simulink model "DC_Drive"  (R2021a)
settings: Solver=VariableStepAuto  StartTime=0.0  StopTime=13  MaxStep=1e-5  RelTol=1e-3
undefined symbols (not defined in the file): sigbuilder_block
libraries: spsMeanLib x6, simulink_extras x5, spsSawtoothGeneratorLib x4, spsTriangleGeneratorLib x2
settings Model: SimulationMode=accelerator  Creator=AHMED  LastModifiedBy=AHMED

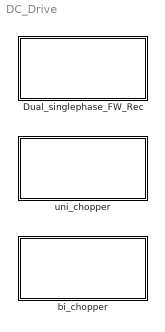
== system DC_Drive ==
  Dual_singlephase_FW_Rec : Subsystem
  bi_chopper : Subsystem
  uni_chopper : Subsystem

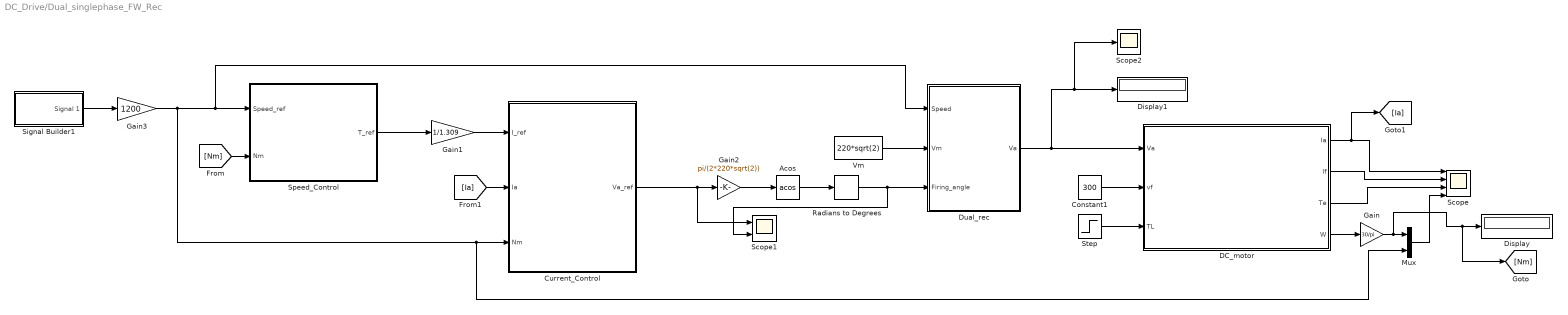
== system DC_Drive/Dual_singlephase_FW_Rec ==
  Acos : Trigonometry  Operator=acos
  Constant1 : Constant  Value=300
  Current_Control : Subsystem
  DC_motor : Subsystem  mask{Ra=0.6, La=12e-3, Rf=240, Lf=120, J=0.05, K=1.309}
  Display : Display
  Display1 : Display
  Dual_rec : Subsystem
  Gain : Gain  Gain=30/pi
  Gain1 : Gain  Gain=1/1.309
  Gain2 : Gain  Gain=pi/(2*220*sqrt(2))
  Gain3 : Gain  Gain=1200
  Mux : Mux  Inputs=2
  Radians to Degrees : simulink_extras/Transformations/Radians to Degrees
  Scope : Scope  NumInputPorts=4
  Scope1 : Scope  NumInputPorts=2
  Scope2 : Scope
  Signal Builder1 : Subsystem  Tag=STV Subsys  LoadFcn=sigbuilder_block('load');  StartFcn=sigbuilder_block('start');  StopFcn=sigbuilder_block('stop');  ClipboardFcn=sigbuilder_block('clipboard');  mask(Sigbuilder block){tuvar=[0:10]}
      mask help: Simulink:masks:SigbuilderBlock_MD
      mask init:
      | if ~strcmp(get_param(bdroot(gcbh),'SimulationStatus'),'stopped') tuvar = sigbuilder_block('maskInit'); end
      settings: CopyFcn=sigbuilder_block('copy');  DeleteFcn=sigbuilder_block('delete');  ModelCloseFcn=sigbuilder_block('modelClose');  PreSaveFcn=sigbuilder_block('preSave');  PauseFcn=sigbuilder_block('pause');  ContinueFcn=sigbuilder_block('continue');  NameChangeFcn=sigbuilder_block('namechange');  OpenFcn=sigbuilder_block('open',[5.4 30 1141.2 522.6 ]);  CloseFcn=sigbuilder_block('close');
      mask Display: plot(0, 0, 100, 100,[2, 2, 32, 32, 2], [68, 8, 8, 68, 68],[32, 2], [38, 38], [32, 19, 2],[53, 60, 44], [32, 17, 17, 2],[16, 16, 31, 31]);txt = getActiveGroup(gcbh);text(2, 100, txt,'verticalAlignment', 'top');
  Speed_Control : Subsystem
  Step : Step  Time=2.25  After=5  SampleTime=0
  Vm : Constant  Value=220*sqrt(2)
  wires:
  Mux/1 -> Scope/4
  Dual_rec/1(Va) -> Scope2/1, Display1/1, DC_motor/1(Va)
  Gain3/1 -> Mux/2, Current_Control/3(Nm), Dual_rec/1(Speed), Speed_Control/1(Speed_ref)
  Current_Control/1(Va_ref) -> Scope1/1, Gain2/1
  Constant1/1 -> DC_motor/2(vf)
  Vm/1 -> Dual_rec/2(Vm)
  DC_motor/2(If) -> Scope/2
  DC_motor/3(Te) -> Scope/3
  Radians to Degrees/1 -> Scope1/2, Dual_rec/3(Firing_angle)
  DC_motor/4(W) -> Gain/1
  Signal Builder1/1(Signal 1) -> Gain3/1
  Gain/1 -> [Nm], Display/1, Mux/1
  DC_motor/1(Ia) -> [Ia], Scope/1
  Acos/1 -> Radians to Degrees/1
  [Nm] -> Speed_Control/2(Nm)
  Speed_Control/1(T_ref) -> Gain1/1
  Gain1/1 -> Current_Control/1(I_ref)
  [Ia] -> Current_Control/2(Ia)
  Step/1 -> DC_motor/3(TL)
  Gain2/1 -> Acos/1

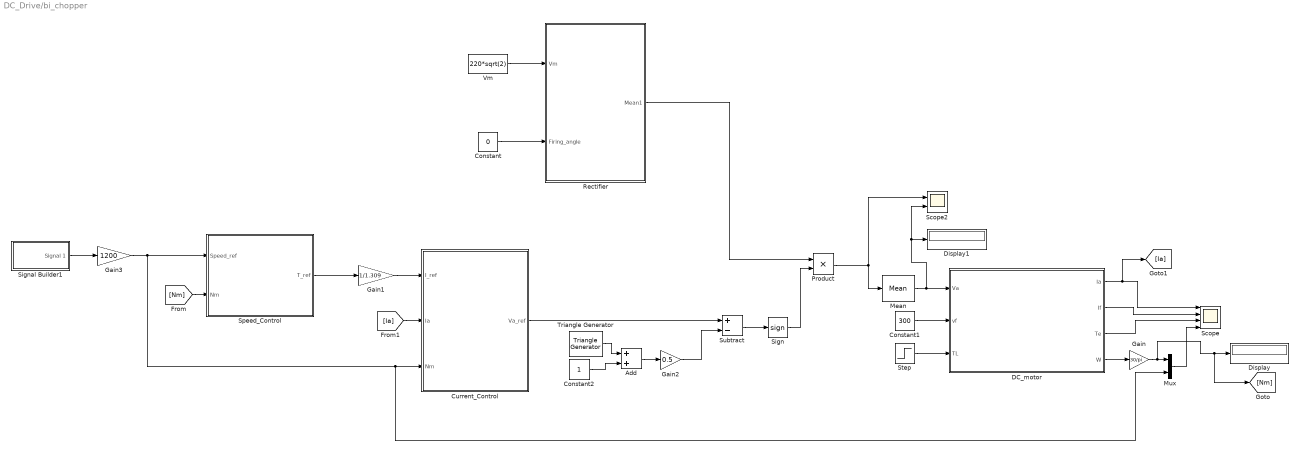
== system DC_Drive/bi_chopper ==
  Add : Sum
  Constant : Constant  Value=0
  Constant1 : Constant  Value=300
  Constant2 : Constant
  Current_Control : Subsystem
  DC_motor : Subsystem  mask{Ra=0.6, La=12e-3, Rf=240, Lf=120, J=0.05, K=1.309}
  Display : Display
  Display1 : Display
  Gain : Gain  Gain=30/pi
  Gain1 : Gain  Gain=1/1.309
  Gain2 : Gain  Gain=0.5
  Gain3 : Gain  Gain=1200
  Mean : spsMeanLib/Mean  Freq=50  Vinit=0  Ts=0
  Mux : Mux  Inputs=2
  Product : Product
  Rectifier : Subsystem
  Scope : Scope  NumInputPorts=4
  Scope2 : Scope  NumInputPorts=2
  Sign : Signum
  Signal Builder1 : Subsystem  Tag=STV Subsys  LoadFcn=sigbuilder_block('load');  StartFcn=sigbuilder_block('start');  StopFcn=sigbuilder_block('stop');  ClipboardFcn=sigbuilder_block('clipboard');  mask(Sigbuilder block){tuvar=[0:10]}
      mask help: Simulink:masks:SigbuilderBlock_MD
      mask init:
      | if ~strcmp(get_param(bdroot(gcbh),'SimulationStatus'),'stopped') tuvar = sigbuilder_block('maskInit'); end
      settings: CopyFcn=sigbuilder_block('copy');  DeleteFcn=sigbuilder_block('delete');  ModelCloseFcn=sigbuilder_block('modelClose');  PreSaveFcn=sigbuilder_block('preSave');  PauseFcn=sigbuilder_block('pause');  ContinueFcn=sigbuilder_block('continue');  NameChangeFcn=sigbuilder_block('namechange');  OpenFcn=sigbuilder_block('open',[5.4 30 1141.2 522.6 ]);  CloseFcn=sigbuilder_block('close');
      mask Display: plot(0, 0, 100, 100,[2, 2, 32, 32, 2], [68, 8, 8, 68, 68],[32, 2], [38, 38], [32, 19, 2],[53, 60, 44], [32, 17, 17, 2],[16, 16, 31, 31]);txt = getActiveGroup(gcbh);text(2, 100, txt,'verticalAlignment', 'top');
  Speed_Control : Subsystem
  Step : Step  Time=2.25  After=5  SampleTime=0
  Subtract : Sum  Inputs=+-
  Triangle Generator : spsTriangleGeneratorLib/Triangle Generator  Freq=1e3  Phase=90  Ts=0
  Vm : Constant  Value=220*sqrt(2)
  wires:
  Mean/1 -> DC_motor/1(Va), Scope2/2, Display1/1
  Add/1 -> Gain2/1
  Constant2/1 -> Add/2
  Triangle Generator/1 -> Add/1
  Constant/1 -> Rectifier/2(Firing_angle)
  Mux/1 -> Scope/4
  Product/1 -> Mean/1, Scope2/1
  Gain3/1 -> Mux/2, Current_Control/3(Nm), Speed_Control/1(Speed_ref)
  Constant1/1 -> DC_motor/2(vf)
  Vm/1 -> Rectifier/1(Vm)
  DC_motor/2(If) -> Scope/2
  DC_motor/3(Te) -> Scope/3
  DC_motor/4(W) -> Gain/1
  Signal Builder1/1(Signal 1) -> Gain3/1
  Gain/1 -> [Nm], Display/1, Mux/1
  DC_motor/1(Ia) -> [Ia], Scope/1
  [Nm] -> Speed_Control/2(Nm)
  Speed_Control/1(T_ref) -> Gain1/1
  Gain1/1 -> Current_Control/1(I_ref)
  [Ia] -> Current_Control/2(Ia)
  Step/1 -> DC_motor/3(TL)
  Current_Control/1(Va_ref) -> Subtract/1
  Gain2/1 -> Subtract/2
  Subtract/1 -> Sign/1
  Rectifier/1(Mean1) -> Product/1
  Sign/1 -> Product/2

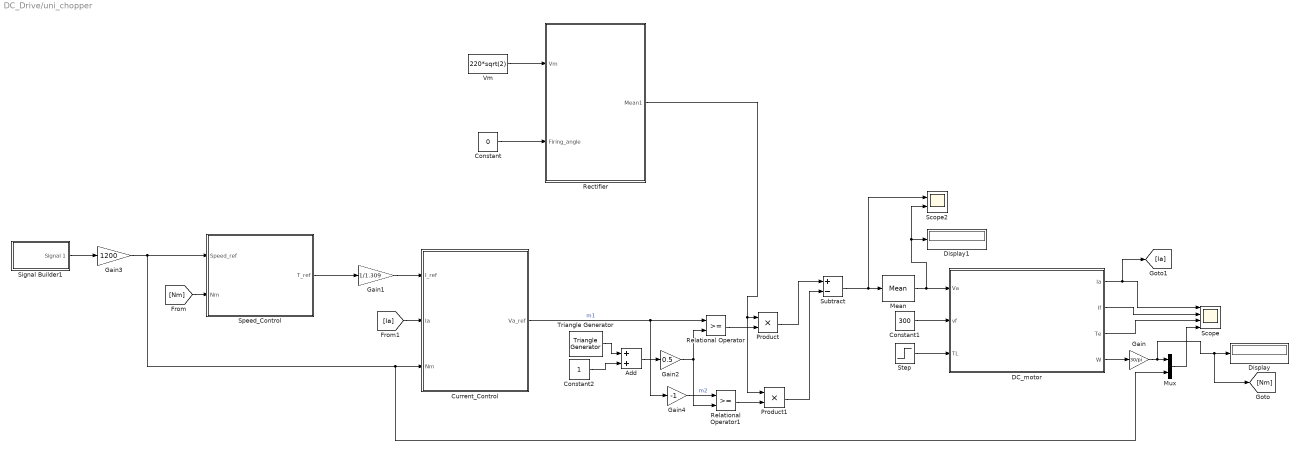
== system DC_Drive/uni_chopper ==
  Add : Sum
  Constant : Constant  Value=0
  Constant1 : Constant  Value=300
  Constant2 : Constant
  Current_Control : Subsystem
  DC_motor : Subsystem  mask{Ra=0.6, La=12e-3, Rf=240, Lf=120, J=0.05, K=1.309}
  Display : Display
  Display1 : Display
  Gain : Gain  Gain=30/pi
  Gain1 : Gain  Gain=1/1.309
  Gain2 : Gain  Gain=0.5
  Gain3 : Gain  Gain=1200
  Gain4 : Gain  Gain=-1
  Mean : spsMeanLib/Mean  Freq=50  Vinit=0  Ts=0
  Mux : Mux  Inputs=2
  Product : Product
  Product1 : Product
  Rectifier : Subsystem
  Relational Operator : RelationalOperator  OutDataTypeStr=boolean  RndMeth=Simplest
  Relational Operator1 : RelationalOperator  OutDataTypeStr=boolean  RndMeth=Simplest
  Scope : Scope  NumInputPorts=4
  Scope2 : Scope  NumInputPorts=2
  Signal Builder1 : Subsystem  Tag=STV Subsys  LoadFcn=sigbuilder_block('load');  StartFcn=sigbuilder_block('start');  StopFcn=sigbuilder_block('stop');  ClipboardFcn=sigbuilder_block('clipboard');  mask(Sigbuilder block){tuvar=[0:10]}
      mask help: Simulink:masks:SigbuilderBlock_MD
      mask init:
      | if ~strcmp(get_param(bdroot(gcbh),'SimulationStatus'),'stopped') tuvar = sigbuilder_block('maskInit'); end
      settings: CopyFcn=sigbuilder_block('copy');  DeleteFcn=sigbuilder_block('delete');  ModelCloseFcn=sigbuilder_block('modelClose');  PreSaveFcn=sigbuilder_block('preSave');  PauseFcn=sigbuilder_block('pause');  ContinueFcn=sigbuilder_block('continue');  NameChangeFcn=sigbuilder_block('namechange');  OpenFcn=sigbuilder_block('open',[5.4 30 1141.2 522.6 ]);  CloseFcn=sigbuilder_block('close');
      mask Display: plot(0, 0, 100, 100,[2, 2, 32, 32, 2], [68, 8, 8, 68, 68],[32, 2], [38, 38], [32, 19, 2],[53, 60, 44], [32, 17, 17, 2],[16, 16, 31, 31]);txt = getActiveGroup(gcbh);text(2, 100, txt,'verticalAlignment', 'top');
  Speed_Control : Subsystem
  Step : Step  Time=2.25  After=5  SampleTime=0
  Subtract : Sum  Inputs=+-
  Triangle Generator : spsTriangleGeneratorLib/Triangle Generator  Freq=1e3  Phase=90  Ts=0
  Vm : Constant  Value=220*sqrt(2)
  wires:
  Step/1 -> DC_motor/3(TL)
  [Ia] -> Current_Control/2(Ia)
  Gain1/1 -> Current_Control/1(I_ref)
  Speed_Control/1(T_ref) -> Gain1/1
  [Nm] -> Speed_Control/2(Nm)
  DC_motor/1(Ia) -> Scope/1, [Ia]
  Gain/1 -> Mux/1, Display/1, [Nm]
  Signal Builder1/1(Signal 1) -> Gain3/1
  DC_motor/4(W) -> Gain/1
  DC_motor/3(Te) -> Scope/3
  DC_motor/2(If) -> Scope/2
  Vm/1 -> Rectifier/1(Vm)
  Constant1/1 -> DC_motor/2(vf)
  Gain3/1 -> Speed_Control/1(Speed_ref), Current_Control/3(Nm), Mux/2
  Subtract/1 -> Scope2/1, Mean/1
  Mux/1 -> Scope/4
  Constant/1 -> Rectifier/2(Firing_angle)
  Triangle Generator/1 -> Add/1
  Constant2/1 -> Add/2
  Add/1 -> Gain2/1
  Current_Control/1(Va_ref) -> Gain4/1, Relational Operator/1  "m1"
  Gain2/1 -> Relational Operator1/2, Relational Operator/2
  Gain4/1 -> Relational Operator1/1  "m2"
  Rectifier/1(Mean1) -> Product1/1, Product/1
  Relational Operator/1 -> Product/2
  Relational Operator1/1 -> Product1/2
  Product/1 -> Subtract/1
  Product1/1 -> Subtract/2
  Mean/1 -> Display1/1, Scope2/2, DC_motor/1(Va)

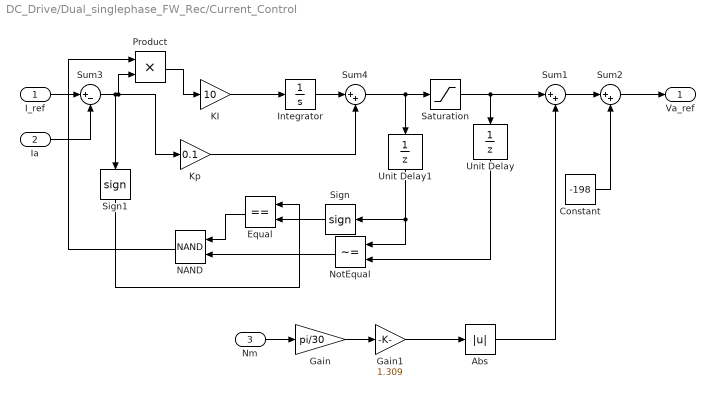
== system DC_Drive/Dual_singlephase_FW_Rec/Current_Control ==
  I_ref : Inport
  Ia : Inport  Port=2
  Nm : Inport  Port=3
  Abs : Abs
  Constant : Constant  Value=-198
  Equal : RelationalOperator  Operator===  OutDataTypeStr=boolean  RndMeth=Simplest
  Gain : Gain  Gain=pi/30
  Gain1 : Gain  Gain=1.309
  Integrator : Integrator
  KI : Gain  Gain=10
  Kp : Gain  Gain=0.1
  NAND : Logic  Operator=NAND  AllPortsSameDT=off  OutDataTypeStr=boolean
  NotEqual : RelationalOperator  Operator=~=  OutDataTypeStr=boolean  RndMeth=Simplest
  Product : Product
  Saturation : Saturate  UpperLimit=198  LowerLimit=-198
  Sign : Signum
  Sign1 : Signum
  Sum1 : Sum  Inputs=|++
  Sum2 : Sum  Inputs=|++
  Sum3 : Sum  Inputs=|+-
  Sum4 : Sum  Inputs=|++
  Unit Delay : UnitDelay  SampleTime=-1  HasFrameUpgradeWarning=on
  Unit Delay1 : UnitDelay  SampleTime=-1  HasFrameUpgradeWarning=on
  Va_ref : Outport
  wires:
  Nm/1 -> Gain/1
  Gain/1 -> Gain1/1
  Gain1/1 -> Abs/1
  Constant/1 -> Sum2/2
  Sum2/1 -> Va_ref/1
  Abs/1 -> Sum1/2
  Integrator/1 -> Sum4/1
  KI/1 -> Integrator/1
  Ia/1 -> Sum3/2
  I_ref/1 -> Sum3/1
  Product/1 -> KI/1
  NotEqual/1 -> NAND/2
  Sum3/1 -> Sign1/1, Kp/1, Product/2
  Saturation/1 -> Sum1/1, Unit Delay/1
  Sign/1 -> Equal/2
  Sign1/1 -> Equal/1
  Unit Delay/1 -> NotEqual/2
  Sum4/1 -> Saturation/1, Unit Delay1/1
  Kp/1 -> Sum4/2
  NAND/1 -> Product/1
  Equal/1 -> NAND/1
  Unit Delay1/1 -> Sign/1, NotEqual/1
  Sum1/1 -> Sum2/1

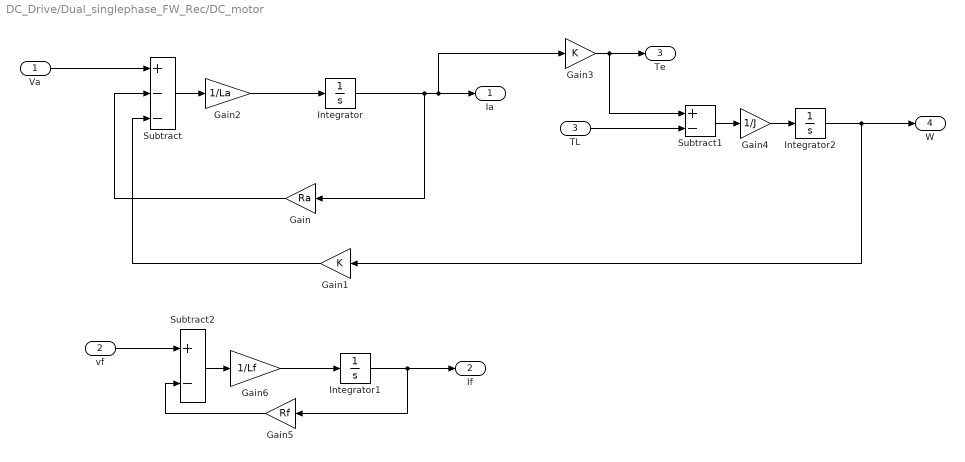
== system DC_Drive/Dual_singlephase_FW_Rec/DC_motor ==
  Va : Inport
  vf : Inport  Port=2
  TL : Inport  Port=3
  Gain : Gain  Gain=Ra
  Gain1 : Gain  Gain=K
  Gain2 : Gain  Gain=1/La
  Gain3 : Gain  Gain=K
  Gain4 : Gain  Gain=1/J
  Gain5 : Gain  Gain=Rf
  Gain6 : Gain  Gain=1/Lf
  Integrator : Integrator
  Integrator1 : Integrator
  Integrator2 : Integrator
  Subtract : Sum  Inputs=+--
  Subtract1 : Sum  Inputs=+-
  Subtract2 : Sum  Inputs=+-
  Ia : Outport
  If : Outport  Port=2
  Te : Outport  Port=3
  W : Outport  Port=4
  wires:
  Gain4/1 -> Integrator2/1
  Gain/1 -> Subtract/2
  Gain2/1 -> Integrator/1
  Gain5/1 -> Subtract2/2
  Subtract2/1 -> Gain6/1
  Subtract/1 -> Gain2/1
  Integrator/1 -> Ia/1, Gain3/1, Gain/1
  Integrator1/1 -> If/1, Gain5/1
  Gain3/1 -> Te/1, Subtract1/1
  Subtract1/1 -> Gain4/1
  TL/1 -> Subtract1/2
  Va/1 -> Subtract/1
  vf/1 -> Subtract2/1
  Gain6/1 -> Integrator1/1
  Gain1/1 -> Subtract/3
  Integrator2/1 -> W/1, Gain1/1

== system DC_Drive/Dual_singlephase_FW_Rec/Dual_rec ==
  Speed : Inport
  Vm : Inport  Port=2
  Firing_angle : Inport  Port=3
  If : If  IfExpression=u1 >= 0
  If Action Subsystem : Subsystem  TreatAsAtomicUnit=on
  If Action Subsystem1 : Subsystem  TreatAsAtomicUnit=on
  Merge : Merge
  Rectifier : Subsystem
  Rectifier1 : Subsystem
  Va : Outport
  wires:
  Rectifier/1(Mean1) -> If Action Subsystem/1(Mean1)
  Rectifier1/1(Mean1) -> If Action Subsystem1/1(Mean1)
  Firing_angle/1 -> Rectifier1/2(Firing_angle), Rectifier/2(Firing_angle)
  Vm/1 -> Rectifier1/1(Vm), Rectifier/1(Vm)
  If/2 -> If Action Subsystem1/Action
  If Action Subsystem/1(Out1) -> Merge/1
  If Action Subsystem1/1(Out1) -> Merge/2
  If/1 -> If Action Subsystem/Action
  Speed/1 -> If/1
  Merge/1 -> Va/1

== system DC_Drive/Dual_singlephase_FW_Rec/Signal Builder1 ==
  Demux : Demux  Tag=STV Demux  Outputs=1
      settings: DisplayOption=none
  FromWs : FromWorkspace  Tag=STV FromWs  VariableName=tuvar
      SigBuilderData=|
      | common.afterFinalStr = 'Extrapolate'
      | common.sampleTime = 0
      | dataSet.timeRange = [0 13]
      | dataSet.name = 'Group 1'
      | sbobj.Groups.Name = 'Group 1'
      | sbobj.Groups.Signals.Name = 'Signal 1'
      | sbobj.Groups.Signals.XData = [0 1 2 3 4 5 8 9 10 11 12 13]
      | sbobj.Groups.Signals.YData = [0 0 0.5 0.5 1 1 -0.5 -0.5 -0.85 -0.85 -0.01 -0.01]
      | sbobj.Groups.TimeRange = [0 13]
  Signal 1 : Outport  Tag=STV Outport
  wires:
  Demux/1 -> Signal 1/1
  FromWs/1 -> Demux/1

== system DC_Drive/Dual_singlephase_FW_Rec/Speed_Control ==
  Speed_ref : Inport
  Nm : Inport  Port=2
  Abs : Abs
  Abs1 : Abs
  Equal : RelationalOperator  Operator===  OutDataTypeStr=boolean  RndMeth=Simplest
  Integrator : Integrator
  KI : Gain  Gain=0.5
  Kp : Gain  Gain=0.5
  NAND : Logic  Operator=NAND  AllPortsSameDT=off  OutDataTypeStr=boolean
  NotEqual : RelationalOperator  Operator=~=  OutDataTypeStr=boolean  RndMeth=Simplest
  Product : Product
  Saturation : Saturate  UpperLimit=(30*746)/(1750*pi/30)  LowerLimit=-(30*746)/(1750*pi/30)
  Sign : Signum
  Sign1 : Signum
  Sum : Sum  Inputs=|+-
  Sum1 : Sum  Inputs=|++
  Unit Delay : UnitDelay  SampleTime=-1  HasFrameUpgradeWarning=on
  Unit Delay1 : UnitDelay  SampleTime=-1  HasFrameUpgradeWarning=on
  T_ref : Outport
  wires:
  Nm/1 -> Abs1/1
  Speed_ref/1 -> Abs/1
  Abs/1 -> Sum/1
  Abs1/1 -> Sum/2
  Sum/1 -> Sign1/1, Kp/1, Product/2
  KI/1 -> Integrator/1
  Kp/1 -> Sum1/2
  Integrator/1 -> Sum1/1
  Sum1/1 -> Saturation/1, Unit Delay1/1
  Saturation/1 -> Unit Delay/1, T_ref/1
  Unit Delay/1 -> NotEqual/2
  Unit Delay1/1 -> Sign/1, NotEqual/1
  NotEqual/1 -> NAND/2
  Sign/1 -> Equal/2
  Sign1/1 -> Equal/1
  Equal/1 -> NAND/1
  NAND/1 -> Product/1
  Product/1 -> KI/1

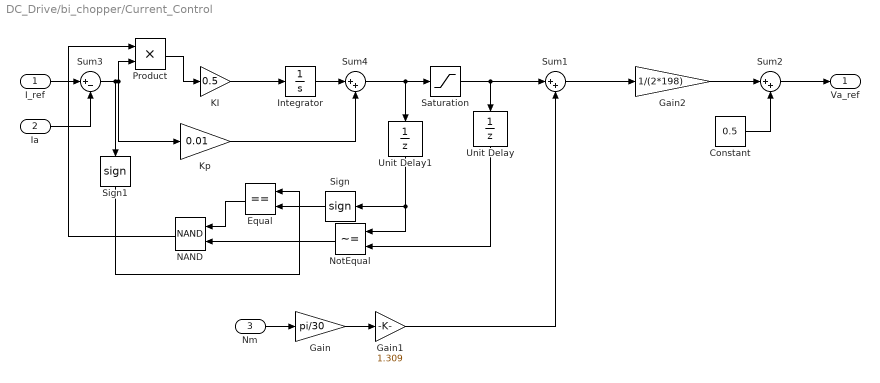
== system DC_Drive/bi_chopper/Current_Control ==
  I_ref : Inport
  Ia : Inport  Port=2
  Nm : Inport  Port=3
  Constant : Constant  Value=0.5
  Equal : RelationalOperator  Operator===  OutDataTypeStr=boolean  RndMeth=Simplest
  Gain : Gain  Gain=pi/30
  Gain1 : Gain  Gain=1.309
  Gain2 : Gain  Gain=1/(2*198)
  Integrator : Integrator
  KI : Gain  Gain=0.5
  Kp : Gain  Gain=0.01
  NAND : Logic  Operator=NAND  AllPortsSameDT=off  OutDataTypeStr=boolean
  NotEqual : RelationalOperator  Operator=~=  OutDataTypeStr=boolean  RndMeth=Simplest
  Product : Product
  Saturation : Saturate  UpperLimit=198*2  LowerLimit=0
  Sign : Signum
  Sign1 : Signum
  Sum1 : Sum  Inputs=|++
  Sum2 : Sum  Inputs=|++
  Sum3 : Sum  Inputs=|+-
  Sum4 : Sum  Inputs=|++
  Unit Delay : UnitDelay  SampleTime=-1  HasFrameUpgradeWarning=on
  Unit Delay1 : UnitDelay  SampleTime=-1  HasFrameUpgradeWarning=on
  Va_ref : Outport
  wires:
  Nm/1 -> Gain/1
  Gain/1 -> Gain1/1
  Sum1/1 -> Gain2/1
  Gain1/1 -> Sum1/2
  Integrator/1 -> Sum4/1
  KI/1 -> Integrator/1
  Ia/1 -> Sum3/2
  I_ref/1 -> Sum3/1
  Product/1 -> KI/1
  NotEqual/1 -> NAND/2
  Sum3/1 -> Sign1/1, Kp/1, Product/2
  Saturation/1 -> Sum1/1, Unit Delay/1
  Sign/1 -> Equal/2
  Sign1/1 -> Equal/1
  Unit Delay/1 -> NotEqual/2
  Sum4/1 -> Saturation/1, Unit Delay1/1
  Kp/1 -> Sum4/2
  NAND/1 -> Product/1
  Equal/1 -> NAND/1
  Unit Delay1/1 -> Sign/1, NotEqual/1
  Gain2/1 -> Sum2/1
  Sum2/1 -> Va_ref/1
  Constant/1 -> Sum2/2

== system DC_Drive/bi_chopper/DC_motor ==
  Va : Inport
  vf : Inport  Port=2
  TL : Inport  Port=3
  Gain : Gain  Gain=Ra
  Gain1 : Gain  Gain=K
  Gain2 : Gain  Gain=1/La
  Gain3 : Gain  Gain=K
  Gain4 : Gain  Gain=1/J
  Gain5 : Gain  Gain=Rf
  Gain6 : Gain  Gain=1/Lf
  Integrator : Integrator
  Integrator1 : Integrator
  Integrator2 : Integrator
  Subtract : Sum  Inputs=+--
  Subtract1 : Sum  Inputs=+-
  Subtract2 : Sum  Inputs=+-
  Ia : Outport
  If : Outport  Port=2
  Te : Outport  Port=3
  W : Outport  Port=4
  wires:
  Gain4/1 -> Integrator2/1
  Gain/1 -> Subtract/2
  Gain2/1 -> Integrator/1
  Gain5/1 -> Subtract2/2
  Subtract2/1 -> Gain6/1
  Subtract/1 -> Gain2/1
  Integrator/1 -> Ia/1, Gain3/1, Gain/1
  Integrator1/1 -> If/1, Gain5/1
  Gain3/1 -> Te/1, Subtract1/1
  Subtract1/1 -> Gain4/1
  TL/1 -> Subtract1/2
  Va/1 -> Subtract/1
  vf/1 -> Subtract2/1
  Gain6/1 -> Integrator1/1
  Gain1/1 -> Subtract/3
  Integrator2/1 -> W/1, Gain1/1

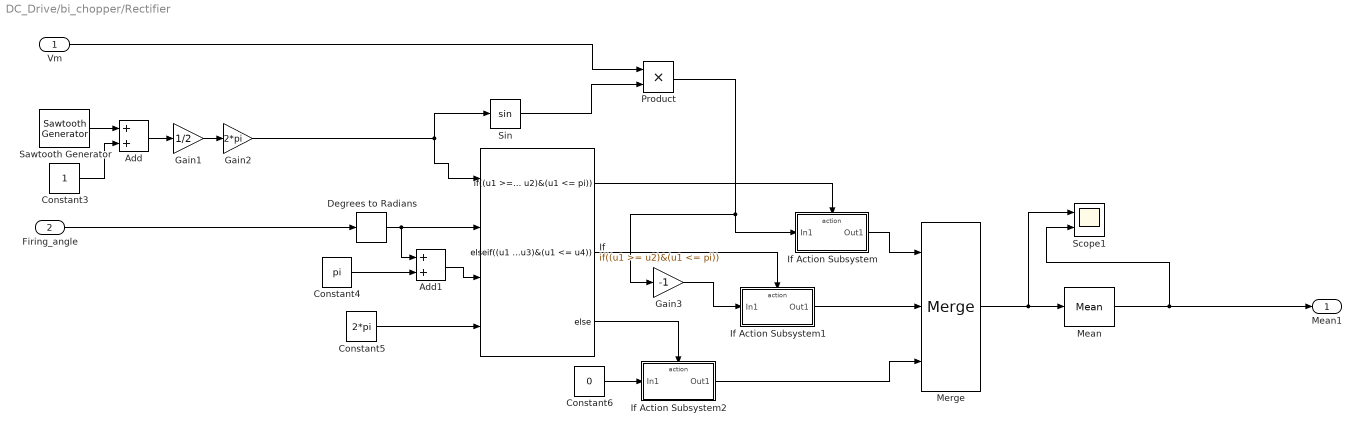
== system DC_Drive/bi_chopper/Rectifier ==
  Vm : Inport
  Firing_angle : Inport  Port=2
  Add : Sum
  Add1 : Sum
  Constant3 : Constant
  Constant4 : Constant  Value=pi
  Constant5 : Constant  Value=2*pi
  Constant6 : Constant  Value=0
  Degrees to Radians : simulink_extras/Transformations/Degrees to Radians
  Gain1 : Gain  Gain=1/2
  Gain2 : Gain  Gain=2*pi
  Gain3 : Gain  Gain=-1
  If : If  NumInputs=4  IfExpression=(u1 >= u2)&(u1 <= pi)  ElseIfExpressions=(u1 >= u3)&(u1 <= u4)
  If Action Subsystem : Subsystem  TreatAsAtomicUnit=on
  If Action Subsystem1 : Subsystem  TreatAsAtomicUnit=on
  If Action Subsystem2 : Subsystem  TreatAsAtomicUnit=on
  Mean : spsMeanLib/Mean  Freq=50  Vinit=0  Ts=0
  Merge : Merge  Inputs=3
  Product : Product
  Sawtooth Generator : spsSawtoothGeneratorLib/Sawtooth Generator  Freq=50  Phase=180  Ts=0
  Scope1 : Scope  NumInputPorts=2
  Sin : Trigonometry
  Mean1 : Outport
  wires:
  Firing_angle/1 -> Degrees to Radians/1
  Mean/1 -> Mean1/1, Scope1/2
  Sin/1 -> Product/2
  If Action Subsystem2/1(Out1) -> Merge/3
  If Action Subsystem/1(Out1) -> Merge/1
  Constant6/1 -> If Action Subsystem2/1(In1)
  Gain3/1 -> If Action Subsystem1/1(In1)
  Gain1/1 -> Gain2/1
  Merge/1 -> Mean/1, Scope1/1
  If/3 -> If Action Subsystem2/Action
  If/2 -> If Action Subsystem1/Action
  Product/1 -> If Action Subsystem/1(In1), Gain3/1
  Constant3/1 -> Add/2
  Constant4/1 -> Add1/2
  Sawtooth Generator/1 -> Add/1
  If Action Subsystem1/1(Out1) -> Merge/2
  Add1/1 -> If/3
  Constant5/1 -> If/4
  Degrees to Radians/1 -> If/2, Add1/1
  Vm/1 -> Product/1
  Gain2/1 -> Sin/1, If/1
  Add/1 -> Gain1/1
  If/1 -> If Action Subsystem/Action

== system DC_Drive/bi_chopper/Signal Builder1 ==
  Demux : Demux  Tag=STV Demux  Outputs=1
      settings: DisplayOption=none
  FromWs : FromWorkspace  Tag=STV FromWs  VariableName=tuvar
      SigBuilderData=|
      | common.afterFinalStr = 'Extrapolate'
      | common.sampleTime = 0
      | dataSet.timeRange = [0 13]
      | dataSet.name = 'Group 1'
      | sbobj.Groups.Name = 'Group 1'
      | sbobj.Groups.Signals.Name = 'Signal 1'
      | sbobj.Groups.Signals.XData = [0 1 2 3 4 5 8 9 10 11 12 13]
      | sbobj.Groups.Signals.YData = [0 0 0.5 0.5 1 1 -0.5 -0.5 -0.85 -0.85 -0.01 -0.01]
      | sbobj.Groups.TimeRange = [0 13]
  Signal 1 : Outport  Tag=STV Outport
  wires:
  Demux/1 -> Signal 1/1
  FromWs/1 -> Demux/1

== system DC_Drive/bi_chopper/Speed_Control ==
  Speed_ref : Inport
  Nm : Inport  Port=2
  Equal : RelationalOperator  Operator===  OutDataTypeStr=boolean  RndMeth=Simplest
  Integrator : Integrator
  KI : Gain  Gain=0.7
  Kp : Gain  Gain=0.5
  NAND : Logic  Operator=NAND  AllPortsSameDT=off  OutDataTypeStr=boolean
  NotEqual : RelationalOperator  Operator=~=  OutDataTypeStr=boolean  RndMeth=Simplest
  Product : Product
  Saturation : Saturate  UpperLimit=(30*746)/(1750*pi/30)  LowerLimit=-(30*746)/(1750*pi/30)
  Sign : Signum
  Sign1 : Signum
  Sum : Sum  Inputs=|+-
  Sum1 : Sum  Inputs=|++
  Unit Delay : UnitDelay  SampleTime=-1  HasFrameUpgradeWarning=on
  Unit Delay1 : UnitDelay  SampleTime=-1  HasFrameUpgradeWarning=on
  T_ref : Outport
  wires:
  Speed_ref/1 -> Sum/1
  Nm/1 -> Sum/2
  Sum/1 -> Sign1/1, Kp/1, Product/2
  KI/1 -> Integrator/1
  Kp/1 -> Sum1/2
  Integrator/1 -> Sum1/1
  Sum1/1 -> Saturation/1, Unit Delay1/1
  Saturation/1 -> Unit Delay/1, T_ref/1
  Unit Delay/1 -> NotEqual/2
  Unit Delay1/1 -> Sign/1, NotEqual/1
  NotEqual/1 -> NAND/2
  Sign/1 -> Equal/2
  Sign1/1 -> Equal/1
  Equal/1 -> NAND/1
  NAND/1 -> Product/1
  Product/1 -> KI/1

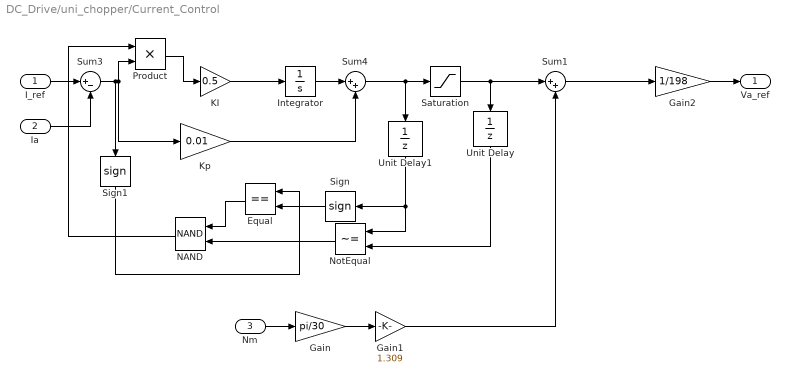
== system DC_Drive/uni_chopper/Current_Control ==
  I_ref : Inport
  Ia : Inport  Port=2
  Nm : Inport  Port=3
  Equal : RelationalOperator  Operator===  OutDataTypeStr=boolean  RndMeth=Simplest
  Gain : Gain  Gain=pi/30
  Gain1 : Gain  Gain=1.309
  Gain2 : Gain  Gain=1/198
  Integrator : Integrator
  KI : Gain  Gain=0.5
  Kp : Gain  Gain=0.01
  NAND : Logic  Operator=NAND  AllPortsSameDT=off  OutDataTypeStr=boolean
  NotEqual : RelationalOperator  Operator=~=  OutDataTypeStr=boolean  RndMeth=Simplest
  Product : Product
  Saturation : Saturate  UpperLimit=198  LowerLimit=-198
  Sign : Signum
  Sign1 : Signum
  Sum1 : Sum  Inputs=|++
  Sum3 : Sum  Inputs=|+-
  Sum4 : Sum  Inputs=|++
  Unit Delay : UnitDelay  SampleTime=-1  HasFrameUpgradeWarning=on
  Unit Delay1 : UnitDelay  SampleTime=-1  HasFrameUpgradeWarning=on
  Va_ref : Outport
  wires:
  Unit Delay1/1 -> NotEqual/1, Sign/1
  Equal/1 -> NAND/1
  NAND/1 -> Product/1
  Kp/1 -> Sum4/2
  Sum4/1 -> Unit Delay1/1, Saturation/1
  Unit Delay/1 -> NotEqual/2
  Sign1/1 -> Equal/1
  Sign/1 -> Equal/2
  Saturation/1 -> Unit Delay/1, Sum1/1
  Sum3/1 -> Product/2, Kp/1, Sign1/1
  NotEqual/1 -> NAND/2
  Product/1 -> KI/1
  I_ref/1 -> Sum3/1
  Ia/1 -> Sum3/2
  KI/1 -> Integrator/1
  Integrator/1 -> Sum4/1
  Gain1/1 -> Sum1/2
  Sum1/1 -> Gain2/1
  Gain/1 -> Gain1/1
  Nm/1 -> Gain/1
  Gain2/1 -> Va_ref/1

== system DC_Drive/uni_chopper/DC_motor ==
  Va : Inport
  vf : Inport  Port=2
  TL : Inport  Port=3
  Gain : Gain  Gain=Ra
  Gain1 : Gain  Gain=K
  Gain2 : Gain  Gain=1/La
  Gain3 : Gain  Gain=K
  Gain4 : Gain  Gain=1/J
  Gain5 : Gain  Gain=Rf
  Gain6 : Gain  Gain=1/Lf
  Integrator : Integrator
  Integrator1 : Integrator
  Integrator2 : Integrator
  Subtract : Sum  Inputs=+--
  Subtract1 : Sum  Inputs=+-
  Subtract2 : Sum  Inputs=+-
  Ia : Outport
  If : Outport  Port=2
  Te : Outport  Port=3
  W : Outport  Port=4
  wires:
  Integrator2/1 -> Gain1/1, W/1
  Gain1/1 -> Subtract/3
  Gain6/1 -> Integrator1/1
  vf/1 -> Subtract2/1
  Va/1 -> Subtract/1
  TL/1 -> Subtract1/2
  Subtract1/1 -> Gain4/1
  Gain3/1 -> Subtract1/1, Te/1
  Integrator1/1 -> Gain5/1, If/1
  Integrator/1 -> Gain/1, Gain3/1, Ia/1
  Subtract/1 -> Gain2/1
  Subtract2/1 -> Gain6/1
  Gain5/1 -> Subtract2/2
  Gain2/1 -> Integrator/1
  Gain/1 -> Subtract/2
  Gain4/1 -> Integrator2/1

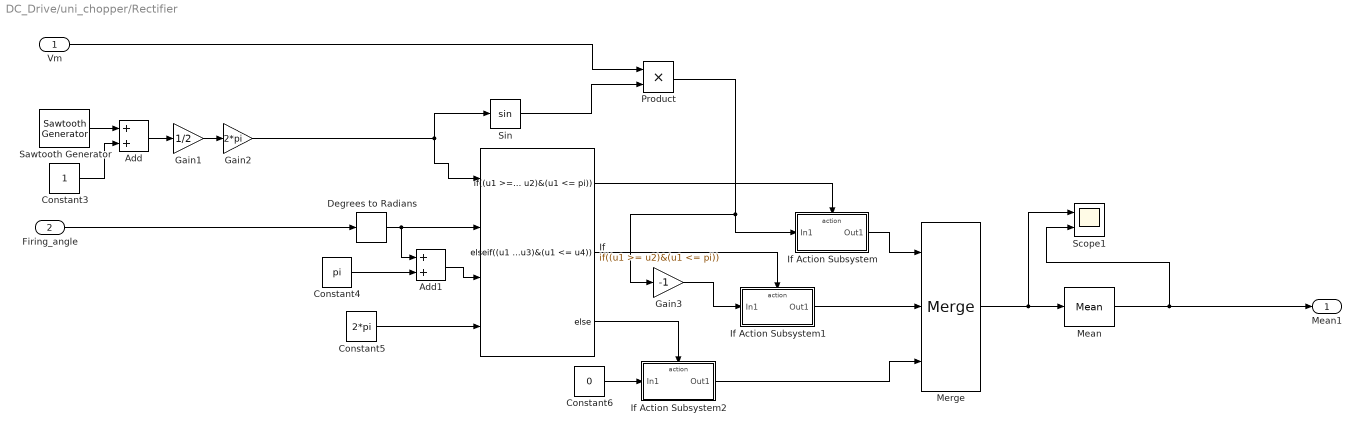
== system DC_Drive/uni_chopper/Rectifier ==
  Vm : Inport
  Firing_angle : Inport  Port=2
  Add : Sum
  Add1 : Sum
  Constant3 : Constant
  Constant4 : Constant  Value=pi
  Constant5 : Constant  Value=2*pi
  Constant6 : Constant  Value=0
  Degrees to Radians : simulink_extras/Transformations/Degrees to Radians
  Gain1 : Gain  Gain=1/2
  Gain2 : Gain  Gain=2*pi
  Gain3 : Gain  Gain=-1
  If : If  NumInputs=4  IfExpression=(u1 >= u2)&(u1 <= pi)  ElseIfExpressions=(u1 >= u3)&(u1 <= u4)
  If Action Subsystem : Subsystem  TreatAsAtomicUnit=on
  If Action Subsystem1 : Subsystem  TreatAsAtomicUnit=on
  If Action Subsystem2 : Subsystem  TreatAsAtomicUnit=on
  Mean : spsMeanLib/Mean  Freq=50  Vinit=0  Ts=0
  Merge : Merge  Inputs=3
  Product : Product
  Sawtooth Generator : spsSawtoothGeneratorLib/Sawtooth Generator  Freq=50  Phase=180  Ts=0
  Scope1 : Scope  NumInputPorts=2
  Sin : Trigonometry
  Mean1 : Outport
  wires:
  If/1 -> If Action Subsystem/Action
  Add/1 -> Gain1/1
  Gain2/1 -> If/1, Sin/1
  Vm/1 -> Product/1
  Degrees to Radians/1 -> Add1/1, If/2
  Constant5/1 -> If/4
  Add1/1 -> If/3
  If Action Subsystem1/1(Out1) -> Merge/2
  Sawtooth Generator/1 -> Add/1
  Constant4/1 -> Add1/2
  Constant3/1 -> Add/2
  Product/1 -> Gain3/1, If Action Subsystem/1(In1)
  If/2 -> If Action Subsystem1/Action
  If/3 -> If Action Subsystem2/Action
  Merge/1 -> Scope1/1, Mean/1
  Gain1/1 -> Gain2/1
  Gain3/1 -> If Action Subsystem1/1(In1)
  Constant6/1 -> If Action Subsystem2/1(In1)
  If Action Subsystem/1(Out1) -> Merge/1
  If Action Subsystem2/1(Out1) -> Merge/3
  Sin/1 -> Product/2
  Mean/1 -> Scope1/2, Mean1/1
  Firing_angle/1 -> Degrees to Radians/1

== system DC_Drive/uni_chopper/Signal Builder1 ==
  Demux : Demux  Tag=STV Demux  Outputs=1
      settings: DisplayOption=none
  FromWs : FromWorkspace  Tag=STV FromWs  VariableName=tuvar
      SigBuilderData=|
      | common.afterFinalStr = 'Extrapolate'
      | common.sampleTime = 0
      | dataSet.timeRange = [0 13]
      | dataSet.name = 'Group 1'
      | sbobj.Groups.Name = 'Group 1'
      | sbobj.Groups.Signals.Name = 'Signal 1'
      | sbobj.Groups.Signals.XData = [0 1 2 3 4 5 8 9 10 11 12 13]
      | sbobj.Groups.Signals.YData = [0 0 0.5 0.5 1 1 -0.5 -0.5 -0.85 -0.85 -0.01 -0.01]
      | sbobj.Groups.TimeRange = [0 13]
  Signal 1 : Outport  Tag=STV Outport
  wires:
  FromWs/1 -> Demux/1
  Demux/1 -> Signal 1/1

== system DC_Drive/uni_chopper/Speed_Control ==
  Speed_ref : Inport
  Nm : Inport  Port=2
  Equal : RelationalOperator  Operator===  OutDataTypeStr=boolean  RndMeth=Simplest
  Integrator : Integrator
  KI : Gain  Gain=0.7
  Kp : Gain  Gain=0.5
  NAND : Logic  Operator=NAND  AllPortsSameDT=off  OutDataTypeStr=boolean
  NotEqual : RelationalOperator  Operator=~=  OutDataTypeStr=boolean  RndMeth=Simplest
  Product : Product
  Saturation : Saturate  UpperLimit=(30*746)/(1750*pi/30)  LowerLimit=-(30*746)/(1750*pi/30)
  Sign : Signum
  Sign1 : Signum
  Sum : Sum  Inputs=|+-
  Sum1 : Sum  Inputs=|++
  Unit Delay : UnitDelay  SampleTime=-1  HasFrameUpgradeWarning=on
  Unit Delay1 : UnitDelay  SampleTime=-1  HasFrameUpgradeWarning=on
  T_ref : Outport
  wires:
  Product/1 -> KI/1
  NAND/1 -> Product/1
  Equal/1 -> NAND/1
  Sign1/1 -> Equal/1
  Sign/1 -> Equal/2
  NotEqual/1 -> NAND/2
  Unit Delay1/1 -> NotEqual/1, Sign/1
  Unit Delay/1 -> NotEqual/2
  Saturation/1 -> T_ref/1, Unit Delay/1
  Sum1/1 -> Unit Delay1/1, Saturation/1
  Integrator/1 -> Sum1/1
  Kp/1 -> Sum1/2
  KI/1 -> Integrator/1
  Sum/1 -> Product/2, Kp/1, Sign1/1
  Nm/1 -> Sum/2
  Speed_ref/1 -> Sum/1

== system DC_Drive/Dual_singlephase_FW_Rec/Dual_rec/If Action Subsystem ==
  Mean1 : Inport
  Action Port : ActionPort  ActionPortLabel=if(u1 >= 0)
  Out1 : Outport
  wires:
  Mean1/1 -> Out1/1

== system DC_Drive/Dual_singlephase_FW_Rec/Dual_rec/If Action Subsystem1 ==
  Mean1 : Inport
  Action Port : ActionPort  ActionPortLabel=else
  Out1 : Outport
  wires:
  Mean1/1 -> Out1/1

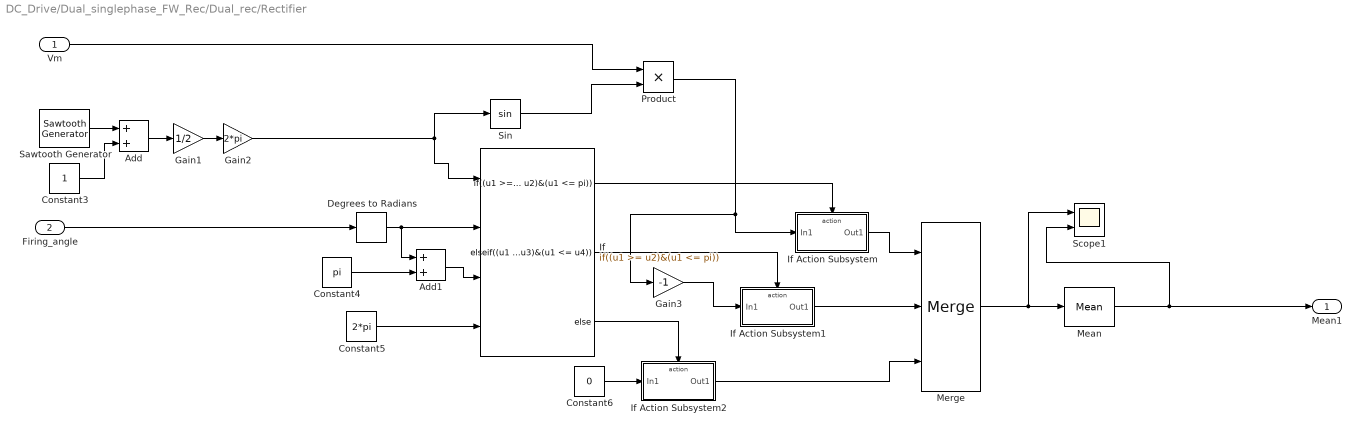
== system DC_Drive/Dual_singlephase_FW_Rec/Dual_rec/Rectifier ==
  Vm : Inport
  Firing_angle : Inport  Port=2
  Add : Sum
  Add1 : Sum
  Constant3 : Constant
  Constant4 : Constant  Value=pi
  Constant5 : Constant  Value=2*pi
  Constant6 : Constant  Value=0
  Degrees to Radians : simulink_extras/Transformations/Degrees to Radians
  Gain1 : Gain  Gain=1/2
  Gain2 : Gain  Gain=2*pi
  Gain3 : Gain  Gain=-1
  If : If  NumInputs=4  IfExpression=(u1 >= u2)&(u1 <= pi)  ElseIfExpressions=(u1 >= u3)&(u1 <= u4)
  If Action Subsystem : Subsystem  TreatAsAtomicUnit=on
  If Action Subsystem1 : Subsystem  TreatAsAtomicUnit=on
  If Action Subsystem2 : Subsystem  TreatAsAtomicUnit=on
  Mean : spsMeanLib/Mean  Freq=50  Vinit=0  Ts=0
  Merge : Merge  Inputs=3
  Product : Product
  Sawtooth Generator : spsSawtoothGeneratorLib/Sawtooth Generator  Freq=50  Phase=180  Ts=0
  Scope1 : Scope  NumInputPorts=2
  Sin : Trigonometry
  Mean1 : Outport
  wires:
  If/1 -> If Action Subsystem/Action
  Add/1 -> Gain1/1
  Gain2/1 -> If/1, Sin/1
  Vm/1 -> Product/1
  Degrees to Radians/1 -> Add1/1, If/2
  Constant5/1 -> If/4
  Add1/1 -> If/3
  If Action Subsystem1/1(Out1) -> Merge/2
  Sawtooth Generator/1 -> Add/1
  Constant4/1 -> Add1/2
  Constant3/1 -> Add/2
  Product/1 -> Gain3/1, If Action Subsystem/1(In1)
  If/2 -> If Action Subsystem1/Action
  If/3 -> If Action Subsystem2/Action
  Merge/1 -> Scope1/1, Mean/1
  Gain1/1 -> Gain2/1
  Gain3/1 -> If Action Subsystem1/1(In1)
  Constant6/1 -> If Action Subsystem2/1(In1)
  If Action Subsystem/1(Out1) -> Merge/1
  If Action Subsystem2/1(Out1) -> Merge/3
  Sin/1 -> Product/2
  Mean/1 -> Scope1/2, Mean1/1
  Firing_angle/1 -> Degrees to Radians/1

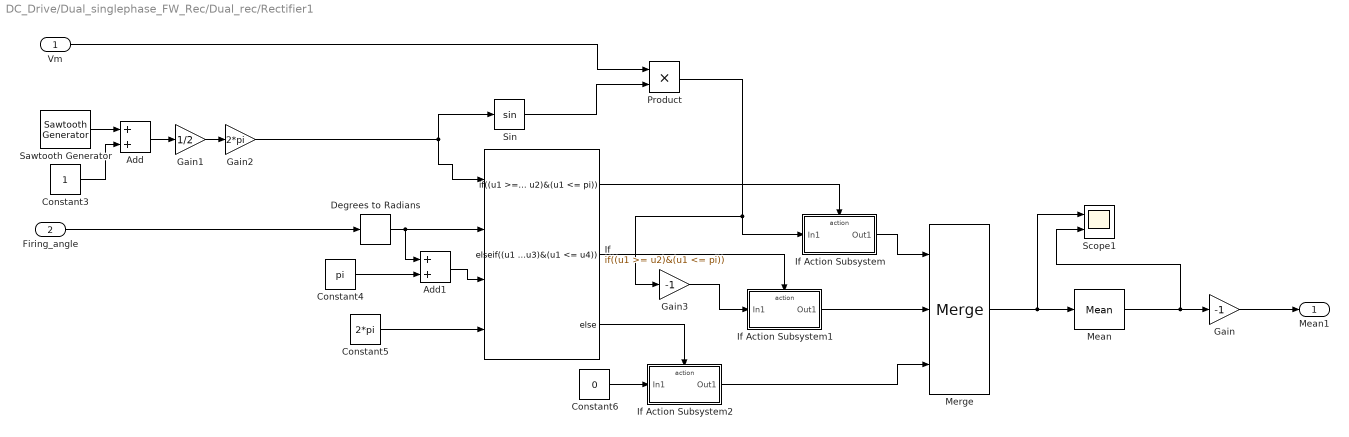
== system DC_Drive/Dual_singlephase_FW_Rec/Dual_rec/Rectifier1 ==
  Vm : Inport
  Firing_angle : Inport  Port=2
  Add : Sum
  Add1 : Sum
  Constant3 : Constant
  Constant4 : Constant  Value=pi
  Constant5 : Constant  Value=2*pi
  Constant6 : Constant  Value=0
  Degrees to Radians : simulink_extras/Transformations/Degrees to Radians
  Gain : Gain  Gain=-1
  Gain1 : Gain  Gain=1/2
  Gain2 : Gain  Gain=2*pi
  Gain3 : Gain  Gain=-1
  If : If  NumInputs=4  IfExpression=(u1 >= u2)&(u1 <= pi)  ElseIfExpressions=(u1 >= u3)&(u1 <= u4)
  If Action Subsystem : Subsystem  TreatAsAtomicUnit=on
  If Action Subsystem1 : Subsystem  TreatAsAtomicUnit=on
  If Action Subsystem2 : Subsystem  TreatAsAtomicUnit=on
  Mean : spsMeanLib/Mean  Freq=50  Vinit=0  Ts=0
  Merge : Merge  Inputs=3
  Product : Product
  Sawtooth Generator : spsSawtoothGeneratorLib/Sawtooth Generator  Freq=50  Phase=180  Ts=0
  Scope1 : Scope  NumInputPorts=2
  Sin : Trigonometry
  Mean1 : Outport
  wires:
  Firing_angle/1 -> Degrees to Radians/1
  Mean/1 -> Gain/1, Scope1/2
  Sin/1 -> Product/2
  If Action Subsystem2/1(Out1) -> Merge/3
  If Action Subsystem/1(Out1) -> Merge/1
  Constant6/1 -> If Action Subsystem2/1(In1)
  Gain3/1 -> If Action Subsystem1/1(In1)
  Gain1/1 -> Gain2/1
  Merge/1 -> Mean/1, Scope1/1
  If/3 -> If Action Subsystem2/Action
  If/2 -> If Action Subsystem1/Action
  Product/1 -> If Action Subsystem/1(In1), Gain3/1
  Constant3/1 -> Add/2
  Constant4/1 -> Add1/2
  Sawtooth Generator/1 -> Add/1
  If Action Subsystem1/1(Out1) -> Merge/2
  Add1/1 -> If/3
  Constant5/1 -> If/4
  Degrees to Radians/1 -> If/2, Add1/1
  Vm/1 -> Product/1
  Gain2/1 -> Sin/1, If/1
  Add/1 -> Gain1/1
  If/1 -> If Action Subsystem/Action
  Gain/1 -> Mean1/1

== system DC_Drive/bi_chopper/Rectifier/If Action Subsystem ==
  In1 : Inport
  Action Port : ActionPort  ActionPortLabel=if((u1 >= u2)&(u1 <= pi))
  Out1 : Outport
  wires:
  In1/1 -> Out1/1

== system DC_Drive/bi_chopper/Rectifier/If Action Subsystem1 ==
  In1 : Inport
  Action Port : ActionPort  ActionPortLabel=elseif((u1 >= u3)&(u1 <= u4))
  Out1 : Outport
  wires:
  In1/1 -> Out1/1

== system DC_Drive/bi_chopper/Rectifier/If Action Subsystem2 ==
  In1 : Inport
  Action Port : ActionPort  ActionPortLabel=else
  Out1 : Outport
  wires:
  In1/1 -> Out1/1

== system DC_Drive/uni_chopper/Rectifier/If Action Subsystem ==
  In1 : Inport
  Action Port : ActionPort  ActionPortLabel=if((u1 >= u2)&(u1 <= pi))
  Out1 : Outport
  wires:
  In1/1 -> Out1/1

== system DC_Drive/uni_chopper/Rectifier/If Action Subsystem1 ==
  In1 : Inport
  Action Port : ActionPort  ActionPortLabel=elseif((u1 >= u3)&(u1 <= u4))
  Out1 : Outport
  wires:
  In1/1 -> Out1/1

== system DC_Drive/uni_chopper/Rectifier/If Action Subsystem2 ==
  In1 : Inport
  Action Port : ActionPort  ActionPortLabel=else
  Out1 : Outport
  wires:
  In1/1 -> Out1/1

== system DC_Drive/Dual_singlephase_FW_Rec/Dual_rec/Rectifier/If Action Subsystem ==
  In1 : Inport
  Action Port : ActionPort  ActionPortLabel=if((u1 >= u2)&(u1 <= pi))
  Out1 : Outport
  wires:
  In1/1 -> Out1/1

== system DC_Drive/Dual_singlephase_FW_Rec/Dual_rec/Rectifier/If Action Subsystem1 ==
  In1 : Inport
  Action Port : ActionPort  ActionPortLabel=elseif((u1 >= u3)&(u1 <= u4))
  Out1 : Outport
  wires:
  In1/1 -> Out1/1

== system DC_Drive/Dual_singlephase_FW_Rec/Dual_rec/Rectifier/If Action Subsystem2 ==
  In1 : Inport
  Action Port : ActionPort  ActionPortLabel=else
  Out1 : Outport
  wires:
  In1/1 -> Out1/1

== system DC_Drive/Dual_singlephase_FW_Rec/Dual_rec/Rectifier1/If Action Subsystem ==
  In1 : Inport
  Action Port : ActionPort  ActionPortLabel=if((u1 >= u2)&(u1 <= pi))
  Out1 : Outport
  wires:
  In1/1 -> Out1/1

== system DC_Drive/Dual_singlephase_FW_Rec/Dual_rec/Rectifier1/If Action Subsystem1 ==
  In1 : Inport
  Action Port : ActionPort  ActionPortLabel=elseif((u1 >= u3)&(u1 <= u4))
  Out1 : Outport
  wires:
  In1/1 -> Out1/1

== system DC_Drive/Dual_singlephase_FW_Rec/Dual_rec/Rectifier1/If Action Subsystem2 ==
  In1 : Inport
  Action Port : ActionPort  ActionPortLabel=else
  Out1 : Outport
  wires:
  In1/1 -> Out1/1
